simulink model "PEMFuelCellSystem_Cathode_cEGR_ExternalMembraneHumidifier_v01"  (R2025b)
settings: Solver=VariableStepAuto  StartTime=0.0  StopTime=100  MaxStep=0.1  RelTol=1e-3  AbsTol=1e-3
model workspace (MAT data in the model file):
  Gas_properties_block = 'PEMFuelCellSystem_Before_v01/Anode_Hydrogen_BOP/Gas Mixture
Properties'
  Gas_properties_candidates : object (value not decoded)
  T_TLU = [223.15 228.15 233.15 238.15 243.15 248.15 253.15 258.15 263.15 268.15 272.66 273.15 ... (115 elements, 1x115)]
  air_control_min_current_A = 3.8
  anode_separator_D = 0.02
  anode_separator_T0 = 20
  anode_separator_area = 0.000314159265359
  anode_separator_dp_nominal = 0.0005
  anode_separator_extra_length = 0.04
  anode_separator_laminar_fraction = 0.001
  anode_separator_length = 0.12
  anode_separator_mdot_nominal = 0.01
  anode_separator_p0 = 0.101325
  anode_separator_roughness = 1.5e-05
  anode_tube_D = 0.02
  cathode_channel_dp_nominal_MPa = 0.0368422
  cathode_channel_flow_area_m2 = 0.00403764556423
  cathode_channel_laminar_fraction = 0.5
  cathode_channel_mdot_nominal_kg_s = 0.27182
  cathode_outlet_chamber_V = 0.2
  cathode_separator_D = 0.05
  cathode_separator_T0 = 20
  cathode_separator_area = 0.00407150407905
  cathode_separator_dp_nominal = 0.002
  cathode_separator_extra_length = 0.05
  cathode_separator_laminar_fraction = 0.001
  cathode_separator_length = 0.15
  cathode_separator_mdot_nominal = 0.40798
  cathode_separator_p0 = 0.101325
  cathode_separator_roughness = 1.5e-05
  cathode_tube_D = 0.05
  cegr_comp_map_t_denom_epsilon = 1e-09
  cegr_cond_tau = 1
  cegr_inlet_mixer_p0 = 0.101325
  cegr_outlet_chamber_p0 = 0.101325
  cegr_pipe_D = 0.072
  cegr_pipe_area = 0.00407150407905
  cegr_pipe_extra_length = 0.1
  cegr_pipe_length = 0.5
  cegr_pipe_p0 = 0.101325
  cegr_pipe_roughness = 1.5e-05
  cegr_valve_max_area = 0.001
  cegr_valve_open_min_area = 1e-10
  comp_inlet_mixer_V = 0.1
  comp_mdot_corr_TLU = [0 0 0 0 0 0.28 0.26 0.24 0.22 0.2 0.56 0.52 ... (15 elements, 5x3)]
  comp_p_ratio_TLU = [1 1.5 2 2.5 3]
  comp_rpm_TLU = [0 50000 80000]
  coolant_num_layers = 20
  coolant_num_passes = 12
  coolant_tube_D = 0.05
  coolant_w_channels = 1
  drive_cycle_current = [0 0 100 100]
  drive_cycle_power = [0 0 40 40]
  drive_cycle_time = [0 0.5 60.5 600]
  drive_cycle_voltage = [427.6 427.6 410 410]
  env_RH = 0.5
  env_T = 20
  env_p = 0.101325
  env_pSat_H2O = 0.00233931818334
  env_yH20 = 0.0115436377169
  env_yO2 = 0.21
  exhaust_bp_valve_control_Ki_area_per_MPa_s = 0.002
  exhaust_bp_valve_max_area = 0.00134
  exhaust_bp_valve_open_min_area = 1e-10
  focused_anode_boundary_T_C = 20
  focused_anode_feed_p_MPa_abs = 0.3
  focused_anode_inlet_mdot_kg_s = 0.008
  focused_anode_inlet_p_MPa_abs = 0.161325
  focused_anode_outlet_p_MPa_abs = 0.101325
  focused_anode_pipe_area = 0.00246300864041
  focused_anode_pipe_extra_length = 0.1
  focused_anode_pipe_length = 1
  focused_anode_pipe_roughness = 1.5e-05
  focused_anode_yH2 = 0.9997
  focused_cathode_inlet_temperature_C = 58.9
  focused_stack_temperature_C = 80
  humidifier_bypass_mode : string (value not decoded)
  intercooler_Dh = 0.05
  intercooler_T0 = 20
  intercooler_area = 0.00785398163397
  intercooler_cond_tau = 1
  intercooler_dp_nominal = 0.005
  intercooler_extra_length = 0.05
  intercooler_laminar_fraction = 0.001
  intercooler_length = 0.25
  intercooler_mdot_nominal = 0.40798
  intercooler_p0 = 0.101325
  intercooler_roughness = 1.5e-05
  membrane_humidifier_dry_area_m2 = 0.01
  membrane_humidifier_dry_extra_length_m = 0.1
  membrane_humidifier_dry_hydraulic_diameter_m = 0.05
  membrane_humidifier_dry_length_m = 1
  membrane_humidifier_dry_roughness_m = 1.5e-05
  membrane_humidifier_heat_conductivity_W_per_m_K = 5
  membrane_humidifier_temperature_transfer_time_constant_s = 0.2
  membrane_humidifier_water_transfer_conductance_kg_s_Pa = 1e-08
  membrane_humidifier_water_transfer_time_constant_s = 0.5
  membrane_humidifier_wet_area_m2 = 0.01
  membrane_humidifier_wet_extra_length_m = 0.1
  membrane_humidifier_wet_hydraulic_diameter_m = 0.05
  membrane_humidifier_wet_length_m = 1
  membrane_humidifier_wet_roughness_m = 1.5e-05
  pSat_H2O_TLU = [0.0039376926592 0.00720321689378 0.0128411282011 0.0223441068076 0.0380050105363 0.0632733889962 0.103238678713 0.165273175188 0.259872929049 0.401739659013 0.586936061043 0.611151401419 ... (115 elements, 1x115)]
  pSat_TLU = [3379.45709837 5023.40410987 1277.63968517 0.0039376926592 3379.45809837 5023.40510987 1277.64068517 0.00720321689378 3379.45909837 5023.40610987 1277.64168517 0.0128411282011 ... (460 elements, 4x115)]
  radiator_H = 0.5
  radiator_L = 1
  radiator_N_fins = 12000
  radiator_N_tubes = 25
  radiator_W = 0.025
  radiator_air_area_fins = 11.5625
  radiator_air_area_primary = 1.223125
  radiator_cp = 910
  radiator_eta_fin = 0.7
  radiator_fin_spacing = 0.002
  radiator_gap_H = 0.0192708333333
  radiator_rho = 2700
  radiator_t_wall = 0.0001
  radiator_tube_H = 0.0015
  radiator_tube_Leq = 2.5
  routeA_air_control_mode_id = 2
  routeA_air_pid_Ki = 0.5
  routeA_air_pid_Kp = 5
  routeA_anode_inlet_pressure_MPa_abs = 0.161325
  routeA_anode_purge_enable = 1
  routeA_anode_purge_off_n2_mole_fraction = 0.1
  routeA_anode_purge_on_n2_mole_fraction = 0.5
  routeA_anode_recirculation_base_command = 0.2
  routeA_anode_recirculation_current_gain_A_inv = 0.00204081632653
  routeA_anode_rh_setpoint = 1
  routeA_backpressure_control_mode_id = 1
  routeA_cathode_humidifier_gain = 1
  routeA_cathode_rh_setpoint = 1
  routeA_cegr_enabled = 1
  routeA_cegr_valve_mode_id = 1
  routeA_command_profile = [0 0.5 60.5 600 0.101325 0.101325 0.101325 0.101325 20 20 20 20 ... (92 elements, 4x23)]
  routeA_command_profile_baseline = [0.101325 20 0.21 0.0115436377169 0.045 3 0.5 0.1613 1 1 0 70 ... (22 elements, 1x22)]
  routeA_command_profile_fields : string (value not decoded)
  routeA_command_profile_schema : string (value not decoded)
  routeA_current_default_ref_A = 28
  routeA_egr_control_Ki_area = 3.92699081699e-05
  routeA_egr_control_Kp_area = 0.000196349540849
  routeA_egr_control_mode_id = 1
  routeA_egr_target_input_mode_id = 1
  routeA_egr_valve_actuator_tau = 0.5
  routeA_egr_valve_area_direct = 3.92699081699e-06
  routeA_external_case_enabled = 0
  routeA_parameter_layer : string (value not decoded)
  routeA_stack_temperature_set_C = 80
  routeA_target_egr_ratio_comp_in = 0.02
  routeA_voltage_current_max_A = 392
  routeA_voltage_current_min_A = 0
  routeA_voltage_default_ref_V = 394.9
  routeA_voltage_pi_Ki = 0.05
  routeA_voltage_pi_Kp = 1
  separator_condensation_enabled = 1
  separator_l2_efficiency = 0.5
  separator_l2_source : string (value not decoded)
  stack_alpha = 1
  stack_area = 380
  stack_iL = 2.5
  stack_io = 2e-14
  stack_mea_cp = 870
  stack_mea_rho = 1800
  stack_num_cells = 606
  stack_num_channels = 8
  stack_t_gdl = 250
  stack_t_membrane = 125
  stack_w_channels = 1.16496474502
  tank_T = 20
  tank_V = 120
  tank_p = 70
  tank_yH2 = 0.9997
libraries: nesl_utility x57, FuelCell_lib x39, fl_lib x24, slpidlib x4
(part 4 of 6)

== system PEMFuelCellSystem_Cathode_cEGR_ExternalMembraneHumidifier_v01/Cathode_Air_Supply_and_cEGR/Cathode_Inlet_Instrumentation ==
  note: Function: in-line cathode inlet instrumentation.
      | Humidity Sensor W -> RH logging; Mass Flow Sensor M_i -> species mass-flow logging. No gas-state source is added here.
  Cathode_Inlet_EnergyFlow_Converter : nesl_utility/PS-Simulink Converter  Description=Convert cathode-inlet mixture energy flow [W] to the named inlet observability chain.  PhysicalDomain=network_engine_domain  SubClassName=ps_output  LeftPortType=input  RightPortType=output  PseudoPeriodic=off  Frequencies=[]  VectorFormat=inherit  Unit=W  AffineConversion=off
  Cathode_Inlet_Humidity_Sensor_FC : FuelCell_lib/sensors/Composition and Humidity Sensor (FC)
      settings: InternalSimscapePortConfiguration="{\"Bottom\":[],\"Left\":[{\"id\":\"A\",\"label\":\"A\",\"type\":\"FuelCell.FuelCell\"}],\"Right\":[{\"id\":\"x_i\",\"label\":\"x_i\",\"type\":\"output\"},{\"id\":\"y_i\",\"label\":\"y_i\",\"type\":\"output\"},{\"id\":\"W\",\"label\":\"W\",\"type\":\"output\"}],\"Top\":[]}"
  Cathode_Inlet_MassFraction_Converter : nesl_utility/PS-Simulink Converter  Description=Convert cathode-inlet sensor mass fractions to the named inlet observability chain.  PhysicalDomain=network_engine_domain  SubClassName=ps_output  LeftPortType=input  RightPortType=output  PseudoPeriodic=off  Frequencies=[]  VectorFormat=inherit  Unit=1  AffineConversion=off
  Cathode_Inlet_Mass_Flow_Sensor_FC : FuelCell_lib/sensors/Mass Flow Rate Sensor (FC)
      settings: InternalSimscapePortConfiguration="{\"Bottom\":[],\"Left\":[{\"id\":\"A\",\"label\":\"A\",\"type\":\"FuelCell.FuelCell\"}],\"Right\":[{\"id\":\"M\",\"label\":\"M\",\"type\":\"output\"},{\"id\":\"Phi_out\",\"label\":\"Phi\",\"type\":\"output\"},{\"id\":\"M_i\",\"label\":\"M_i\",\"type\":\"output\"},{\"id\":\"B\",\"label\":\"B\",\"type\":\"FuelCell.FuelCell\"}],\"Top\":[]}"
  Cathode_Inlet_Mdot_Converter : nesl_utility/PS-Simulink Converter  Description=Convert cathode-inlet total mass flow [kg/s] to the named inlet observability chain.  PhysicalDomain=network_engine_domain  SubClassName=ps_output  LeftPortType=input  RightPortType=output  PseudoPeriodic=off  Frequencies=[]  VectorFormat=inherit  Unit=kg/s  AffineConversion=off
  Cathode_Inlet_MoleFraction_Converter : nesl_utility/PS-Simulink Converter  Description=Convert cathode-inlet sensor mole fractions to the named inlet observability chain.  PhysicalDomain=network_engine_domain  SubClassName=ps_output  LeftPortType=input  RightPortType=output  PseudoPeriodic=off  Frequencies=[]  VectorFormat=inherit  Unit=1  AffineConversion=off
  Inlet_Result_Observability : Subsystem  Description=Records cathode-inlet relative humidity and species mass-flow vector for the V-SH result contract.
  cathode_air_from_bop : PMIOPort  Side=Left
  cathode_air_to_stack : PMIOPort  Port=2  Side=Right
  wires:
  Cathode_Inlet_MassFraction_Converter/1 -> Inlet_Result_Observability/1(inlet_mass_fraction)  "routeA_xi_ca_in_sensor"
  Cathode_Inlet_MoleFraction_Converter/1 -> Inlet_Result_Observability/2(inlet_mole_fraction)  "routeA_yi_ca_in_sensor"
  Cathode_Inlet_Mdot_Converter/1 -> Inlet_Result_Observability/3(inlet_mdot_kg_s)  "routeA_mdot_ca_in"
  Cathode_Inlet_EnergyFlow_Converter/1 -> Inlet_Result_Observability/4(inlet_energy_flow_W)  "routeA_energy_flow_ca_in_W"
  connections:
  Cathode_Inlet_Mass_Flow_Sensor_FC/RConn2 -- Cathode_Inlet_EnergyFlow_Converter/LConn1
  Cathode_Inlet_Humidity_Sensor_FC/RConn2 -- Cathode_Inlet_MoleFraction_Converter/LConn1
  Cathode_Inlet_Humidity_Sensor_FC/LConn1 -- Cathode_Inlet_Mass_Flow_Sensor_FC/LConn1 -- cathode_air_from_bop/RConn1
  Cathode_Inlet_Mass_Flow_Sensor_FC/RConn3 -- Inlet_Result_Observability/LConn2
  Cathode_Inlet_Mass_Flow_Sensor_FC/RConn1 -- Cathode_Inlet_Mdot_Converter/LConn1
  Cathode_Inlet_Humidity_Sensor_FC/RConn3 -- Inlet_Result_Observability/LConn1
  Cathode_Inlet_Humidity_Sensor_FC/RConn1 -- Cathode_Inlet_MassFraction_Converter/LConn1
  Cathode_Inlet_Mass_Flow_Sensor_FC/RConn4 -- cathode_air_to_stack/RConn1

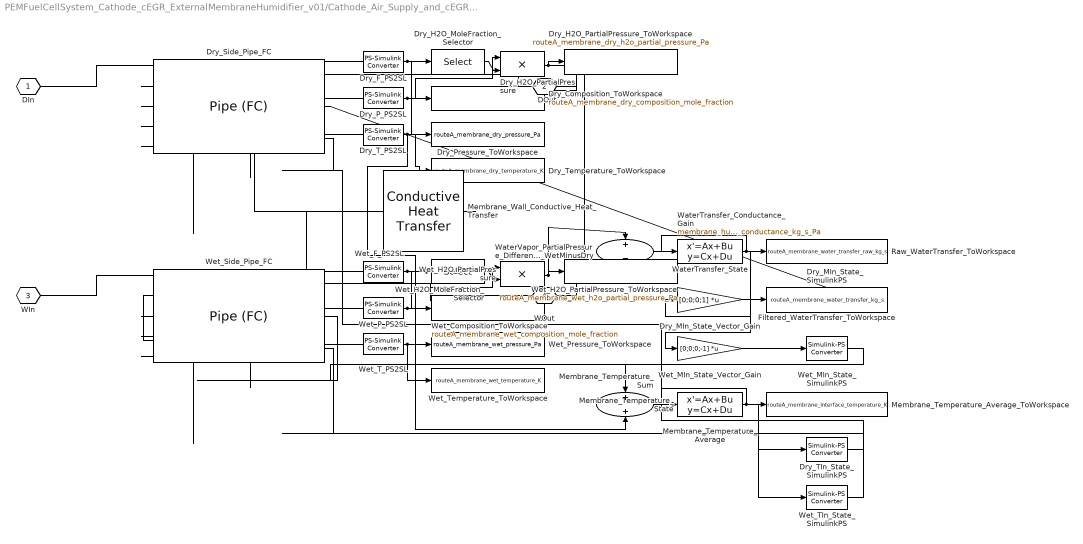
== system PEMFuelCellSystem_Cathode_cEGR_ExternalMembraneHumidifier_v01/Cathode_Air_Supply_and_cEGR/Cathode_Membrane_Humidifier ==
  Dry_Composition_ToWorkspace : ToWorkspace  VariableName=routeA_membrane_dry_composition_mole_fraction  SaveFormat=Structure With Time  SampleTime=-1
  Dry_F_PS2SL : nesl_utility/PS-Simulink Converter  PhysicalDomain=network_engine_domain  SubClassName=ps_output  LeftPortType=input  RightPortType=output  PseudoPeriodic=off  Frequencies=[]  VectorFormat=inherit  Unit=1  AffineConversion=off
  Dry_H2O_MoleFraction_Selector : Selector  InputPortWidth=4  IndexOptions=Index vector (dialog)  Indices=4  OutputSizes=1
  Dry_H2O_PartialPressure : Product  Inputs=**
  Dry_H2O_PartialPressure_ToWorkspace : ToWorkspace  VariableName=routeA_membrane_dry_h2o_partial_pressure_Pa  SaveFormat=Structure With Time  SampleTime=-1
  Dry_MIn_State_SimulinkPS : nesl_utility/Simulink-PS Converter  PhysicalDomain=network_engine_domain  SubClassName=ps_input  LeftPortType=input  RightPortType=output  PseudoPeriodic=off  Frequencies=[]  NoiseDistribution=none  NoiseParameters=[]  Unit=kg/s  AffineConversion=off  FilteringAndDerivatives=provide  SimscapeFilterOrder=1  InputFilterTimeConstant=0.001  UdotUserProvided=0
  Dry_MIn_State_Vector_Gain : Gain  Gain=[0;0;0;1]  Multiplication=Matrix(K*u)
  Dry_P_PS2SL : nesl_utility/PS-Simulink Converter  PhysicalDomain=network_engine_domain  SubClassName=ps_output  LeftPortType=input  RightPortType=output  PseudoPeriodic=off  Frequencies=[]  VectorFormat=inherit  Unit=Pa  AffineConversion=off
  Dry_Pressure_ToWorkspace : ToWorkspace  VariableName=routeA_membrane_dry_pressure_Pa  SaveFormat=Structure With Time  SampleTime=-1
  Dry_Side_Pipe_FC : FuelCell_lib/elements/Pipe (FC)  length=membrane_humidifier_dry_length_m m  area=membrane_humidifier_dry_area_m2 m^2  Dh=membrane_humidifier_dry_hydraulic_diameter_m m  extra_length=membrane_humidifier_dry_extra_length_m m  roughness=membrane_humidifier_dry_roughness_m m  Re_lam=2000  Re_tur=4000  shape_factor=64  Nu_lam=3.66  tau_c=cegr_cond_tau s  isCond=[0;0;0;0]  volMeas=true  compMeas=FuelCell.enum.Composition.Mole  p0=env_p MPa  T0=focused_cathode_inlet_temperature_C degC  comp=FuelCell.enum.Composition.Mole  y0=[1-env_yO2-env_yH20; env_yO2; 0; env_yH20]  x0=[1;0;0;0]
      settings: InternalSimscapePortConfiguration="{\"Bottom\":[{\"id\":\"MIn\",\"label\":\"M_in\",\"type\":\"input\"},{\"id\":\"TIn\",\"label\":\"T_in\",\"type\":\"input\"}],\"Left\":[{\"id\":\"A\",\"label\":\"A\",\"type\":\"FuelCell.FuelCell\"},{\"id\":\"H\",\"label\":\"H\",\"type\":\"foundation.thermal.thermal\"}],\"Right\":[{\"id\":\"B\",\"label\":\"B\",\"type\":\"FuelCell.FuelCell\"}],\"Top\":[{\"id\":\"F\",\"label\":\"F\",\"type\":\"output\"},{\"id\":\"p\",\"label\":\"p\",\"type\":\"output\"},{\"id\":\"T\",\"label\":\"T\",\"type\":\"output\"}]}"
  Dry_TIn_State_SimulinkPS : nesl_utility/Simulink-PS Converter  PhysicalDomain=network_engine_domain  SubClassName=ps_input  LeftPortType=input  RightPortType=output  PseudoPeriodic=off  Frequencies=[]  NoiseDistribution=none  NoiseParameters=[]  Unit=K  AffineConversion=off  FilteringAndDerivatives=provide  SimscapeFilterOrder=1  InputFilterTimeConstant=0.001  UdotUserProvided=0
  Dry_T_PS2SL : nesl_utility/PS-Simulink Converter  PhysicalDomain=network_engine_domain  SubClassName=ps_output  LeftPortType=input  RightPortType=output  PseudoPeriodic=off  Frequencies=[]  VectorFormat=inherit  Unit=K  AffineConversion=off
  Dry_Temperature_ToWorkspace : ToWorkspace  VariableName=routeA_membrane_dry_temperature_K  SaveFormat=Structure With Time  SampleTime=-1
  Filtered_WaterTransfer_ToWorkspace : ToWorkspace  VariableName=routeA_membrane_water_transfer_kg_s  SaveFormat=Structure With Time  SampleTime=-1
  Membrane_Temperature_Average : Gain  Gain=0.5
  Membrane_Temperature_Average_ToWorkspace : ToWorkspace  VariableName=routeA_membrane_interface_temperature_K  SaveFormat=Structure With Time  SampleTime=-1
  Membrane_Temperature_State : StateSpace  A=-1/membrane_humidifier_temperature_transfer_time_constant_s  B=1/membrane_humidifier_temperature_transfer_time_constant_s  D=0  InitialCondition=env_T+273.15
  Membrane_Temperature_Sum : Sum
  Membrane_Wall_Conductive_Heat_Transfer : fl_lib/Thermal/Thermal Elements/Conductive Heat Transfer  thermal_type=foundation.enum.ConstantVariableTabulated.Constant  wall_geometry=foundation.enum.ConductionWallGeometry.Planar  area=1 m^2  thickness=1 m  d_in=0.05 m  d_out=0.1 m  L=1 m  th_cond_min=10 W/(K*m)  th_cond=membrane_humidifier_heat_conductivity_W_per_m_K W/(K*m)  th_cond_TLU=[413, 401, 392, 383, 371, 357, 342] W/(K*m)  temp_TLU=[200, 273, 400, 600, 800, 1000, 1200] K  T_specify=off  T_priority=None  T=0 K  T_nominal_specify=off  T_nominal_value=1  T_nominal_unit=K  Q_specify=off  Q_priority=None  Q=0 W  Q_nominal_specify=off  Q_nominal_value=1  Q_nominal_unit=W
  Raw_WaterTransfer_ToWorkspace : ToWorkspace  VariableName=routeA_membrane_water_transfer_raw_kg_s  SaveFormat=Structure With Time  SampleTime=-1
  WaterTransfer_Conductance_Gain : Gain  Gain=membrane_humidifier_water_transfer_conductance_kg_s_Pa
  WaterTransfer_State : StateSpace  A=-1/membrane_humidifier_water_transfer_time_constant_s  B=1/membrane_humidifier_water_transfer_time_constant_s  D=0  InitialCondition=0
  WaterVapor_PartialPressure_Difference_WetMinusDry : Sum  Inputs=+-
  Wet_Composition_ToWorkspace : ToWorkspace  VariableName=routeA_membrane_wet_composition_mole_fraction  SaveFormat=Structure With Time  SampleTime=-1
  Wet_F_PS2SL : nesl_utility/PS-Simulink Converter  PhysicalDomain=network_engine_domain  SubClassName=ps_output  LeftPortType=input  RightPortType=output  PseudoPeriodic=off  Frequencies=[]  VectorFormat=inherit  Unit=1  AffineConversion=off
  Wet_H2O_MoleFraction_Selector : Selector  InputPortWidth=4  IndexOptions=Index vector (dialog)  Indices=4  OutputSizes=1
  Wet_H2O_PartialPressure : Product  Inputs=**
  Wet_H2O_PartialPressure_ToWorkspace : ToWorkspace  VariableName=routeA_membrane_wet_h2o_partial_pressure_Pa  SaveFormat=Structure With Time  SampleTime=-1
  Wet_MIn_State_SimulinkPS : nesl_utility/Simulink-PS Converter  PhysicalDomain=network_engine_domain  SubClassName=ps_input  LeftPortType=input  RightPortType=output  PseudoPeriodic=off  Frequencies=[]  NoiseDistribution=none  NoiseParameters=[]  Unit=kg/s  AffineConversion=off  FilteringAndDerivatives=provide  SimscapeFilterOrder=1  InputFilterTimeConstant=0.001  UdotUserProvided=0
  Wet_MIn_State_Vector_Gain : Gain  Gain=[0;0;0;-1]  Multiplication=Matrix(K*u)
  Wet_P_PS2SL : nesl_utility/PS-Simulink Converter  PhysicalDomain=network_engine_domain  SubClassName=ps_output  LeftPortType=input  RightPortType=output  PseudoPeriodic=off  Frequencies=[]  VectorFormat=inherit  Unit=Pa  AffineConversion=off
  Wet_Pressure_ToWorkspace : ToWorkspace  VariableName=routeA_membrane_wet_pressure_Pa  SaveFormat=Structure With Time  SampleTime=-1
  Wet_Side_Pipe_FC : FuelCell_lib/elements/Pipe (FC)  length=membrane_humidifier_wet_length_m m  area=membrane_humidifier_wet_area_m2 m^2  Dh=membrane_humidifier_wet_hydraulic_diameter_m m  extra_length=membrane_humidifier_wet_extra_length_m m  roughness=membrane_humidifier_wet_roughness_m m  Re_lam=2000  Re_tur=4000  shape_factor=64  Nu_lam=3.66  tau_c=cegr_cond_tau s  isCond=[0;0;0;0]  volMeas=true  compMeas=FuelCell.enum.Composition.Mole  p0=cegr_outlet_chamber_p0 MPa  T0=env_T degC  comp=FuelCell.enum.Composition.Mole  y0=[1-env_yO2-env_yH20; env_yO2; 0; env_yH20]  x0=[1-env_yO2-env_yH20; env_yO2; 0; env_yH20]
      settings: InternalSimscapePortConfiguration="{\"Bottom\":[{\"id\":\"MIn\",\"label\":\"M_in\",\"type\":\"input\"},{\"id\":\"TIn\",\"label\":\"T_in\",\"type\":\"input\"}],\"Left\":[{\"id\":\"A\",\"label\":\"A\",\"type\":\"FuelCell.FuelCell\"},{\"id\":\"H\",\"label\":\"H\",\"type\":\"foundation.thermal.thermal\"}],\"Right\":[{\"id\":\"B\",\"label\":\"B\",\"type\":\"FuelCell.FuelCell\"}],\"Top\":[{\"id\":\"F\",\"label\":\"F\",\"type\":\"output\"},{\"id\":\"p\",\"label\":\"p\",\"type\":\"output\"},{\"id\":\"T\",\"label\":\"T\",\"type\":\"output\"}]}"
  Wet_TIn_State_SimulinkPS : nesl_utility/Simulink-PS Converter  PhysicalDomain=network_engine_domain  SubClassName=ps_input  LeftPortType=input  RightPortType=output  PseudoPeriodic=off  Frequencies=[]  NoiseDistribution=none  NoiseParameters=[]  Unit=K  AffineConversion=off  FilteringAndDerivatives=provide  SimscapeFilterOrder=1  InputFilterTimeConstant=0.001  UdotUserProvided=0
  Wet_T_PS2SL : nesl_utility/PS-Simulink Converter  PhysicalDomain=network_engine_domain  SubClassName=ps_output  LeftPortType=input  RightPortType=output  PseudoPeriodic=off  Frequencies=[]  VectorFormat=inherit  Unit=K  AffineConversion=off
  Wet_Temperature_ToWorkspace : ToWorkspace  VariableName=routeA_membrane_wet_temperature_K  SaveFormat=Structure With Time  SampleTime=-1
  DIn : PMIOPort  Side=Left
  DOut : PMIOPort  Port=2  Side=Right
  WIn : PMIOPort  Port=3  Side=Left
  WOut : PMIOPort  Port=4  Side=Right
  wires:
  Dry_F_PS2SL/1 -> Dry_H2O_MoleFraction_Selector/1, Dry_Composition_ToWorkspace/1
  Dry_P_PS2SL/1 -> Dry_H2O_PartialPressure/1, Dry_Pressure_ToWorkspace/1
  Dry_T_PS2SL/1 -> Dry_Temperature_ToWorkspace/1, Membrane_Temperature_Sum/1
  Dry_H2O_MoleFraction_Selector/1 -> Dry_H2O_PartialPressure/2
  Dry_H2O_PartialPressure/1 -> Dry_H2O_PartialPressure_ToWorkspace/1, WaterVapor_PartialPressure_Difference_WetMinusDry/2
  Wet_F_PS2SL/1 -> Wet_H2O_MoleFraction_Selector/1, Wet_Composition_ToWorkspace/1
  Wet_P_PS2SL/1 -> Wet_Pressure_ToWorkspace/1, Wet_H2O_PartialPressure/1
  Wet_T_PS2SL/1 -> Wet_Temperature_ToWorkspace/1, Membrane_Temperature_Sum/2
  Wet_H2O_MoleFraction_Selector/1 -> Wet_H2O_PartialPressure/2
  Wet_H2O_PartialPressure/1 -> Wet_H2O_PartialPressure_ToWorkspace/1, WaterVapor_PartialPressure_Difference_WetMinusDry/1
  WaterVapor_PartialPressure_Difference_WetMinusDry/1 -> WaterTransfer_Conductance_Gain/1
  Membrane_Temperature_Sum/1 -> Membrane_Temperature_Average/1
  Dry_MIn_State_Vector_Gain/1 -> Dry_MIn_State_SimulinkPS/1
  Wet_MIn_State_Vector_Gain/1 -> Wet_MIn_State_SimulinkPS/1
  WaterTransfer_State/1 -> Filtered_WaterTransfer_ToWorkspace/1, Dry_MIn_State_Vector_Gain/1, Wet_MIn_State_Vector_Gain/1
  Membrane_Temperature_State/1 -> Dry_TIn_State_SimulinkPS/1, Wet_TIn_State_SimulinkPS/1
  WaterTransfer_Conductance_Gain/1 -> WaterTransfer_State/1, Raw_WaterTransfer_ToWorkspace/1
  Membrane_Temperature_Average/1 -> Membrane_Temperature_State/1, Membrane_Temperature_Average_ToWorkspace/1
  connections:
  DIn/RConn1 -- Dry_Side_Pipe_FC/LConn1
  Dry_Side_Pipe_FC/RConn1 -- DOut/RConn1
  WIn/RConn1 -- Wet_Side_Pipe_FC/LConn1
  Wet_Side_Pipe_FC/RConn1 -- WOut/RConn1
  Membrane_Wall_Conductive_Heat_Transfer/RConn1 -- Wet_Side_Pipe_FC/LConn2
  Dry_Side_Pipe_FC/LConn3 -- Dry_F_PS2SL/LConn1
  Dry_Side_Pipe_FC/LConn4 -- Dry_P_PS2SL/LConn1
  Dry_Side_Pipe_FC/LConn5 -- Dry_T_PS2SL/LConn1
  Wet_Side_Pipe_FC/LConn3 -- Wet_F_PS2SL/LConn1
  Wet_Side_Pipe_FC/LConn4 -- Wet_P_PS2SL/LConn1
  Wet_Side_Pipe_FC/LConn5 -- Wet_T_PS2SL/LConn1
  Dry_Side_Pipe_FC/LConn2 -- Membrane_Wall_Conductive_Heat_Transfer/LConn1
  Wet_TIn_State_SimulinkPS/RConn1 -- Wet_Side_Pipe_FC/RConn3
  Wet_MIn_State_SimulinkPS/RConn1 -- Wet_Side_Pipe_FC/RConn2
  Dry_TIn_State_SimulinkPS/RConn1 -- Dry_Side_Pipe_FC/RConn3
  Dry_MIn_State_SimulinkPS/RConn1 -- Dry_Side_Pipe_FC/RConn2

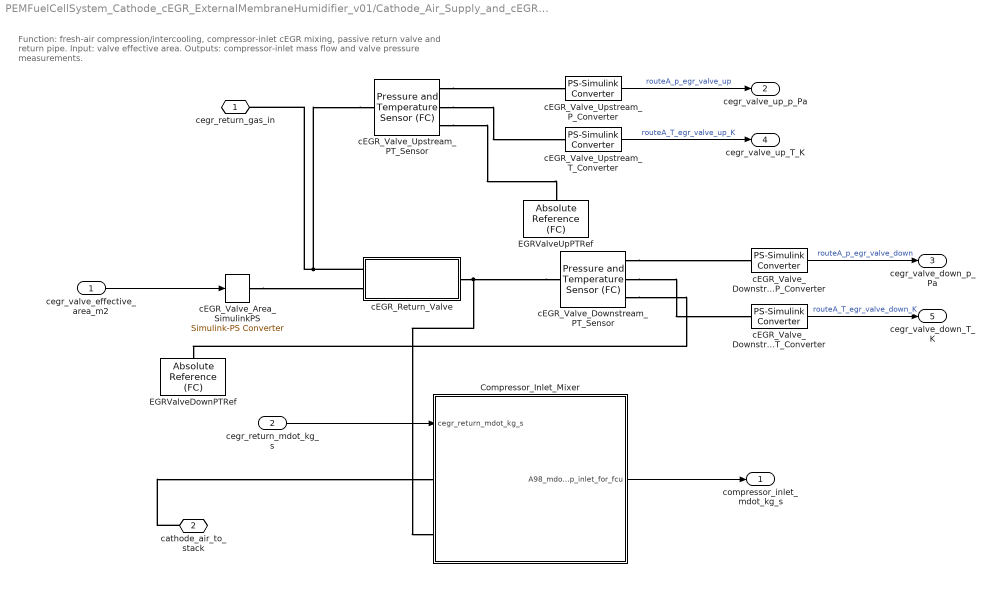
== system PEMFuelCellSystem_Cathode_cEGR_ExternalMembraneHumidifier_v01/Cathode_Air_Supply_and_cEGR/Fresh_Air_Compression_and_cEGR ==
  note: Function: fresh-air compression/intercooling, compressor-inlet cEGR mixing, passive return valve and return pipe.
      | Input: valve effective area. Outputs: compressor-inlet mass flow and valve pressure measurements.
  cegr_valve_effective_area_m2 : Inport
  cegr_return_mdot_kg_s : Inport  Port=2
  Compressor_Inlet_Mixer : Subsystem  Tag=PublishSubsystem  Description=Fresh-air boundary, compressor and intercooler path with compressor-inlet cEGR mixing. External humidifier injection is disabled for V-SH.
      mask Display:
      | plot(0, 0)
      | plot(100, 100)
      | 
      | n = 80;
      | r1 = 15;
      | r2 = 30;
      | 
      | plot(cos(linspace(0, 2*pi, n))*r1 + 65, sin(linspace(0, 2*pi, n))*r1 + 50)
      | plot(cos(linspace(0, 2*pi, n))*r2 + 65, sin(linspace(0, 2*pi, n))*r2 + 50)
      | 
      | plot([65 30 30 42], [80 80 70 70])
  EGRValveDownPTRef : FuelCell_lib/elements/Absolute Reference (FC)
      settings: InternalSimscapePortConfiguration="{\"Bottom\":[],\"Left\":[{\"id\":\"A\",\"label\":\"\",\"type\":\"FuelCell.FuelCell\"}],\"Right\":[],\"Top\":[]}"
  EGRValveUpPTRef : FuelCell_lib/elements/Absolute Reference (FC)
      settings: InternalSimscapePortConfiguration="{\"Bottom\":[],\"Left\":[{\"id\":\"A\",\"label\":\"\",\"type\":\"FuelCell.FuelCell\"}],\"Right\":[],\"Top\":[]}"
  cEGR_Return_Valve : Subsystem  Variant=on
  cEGR_Valve_Area_SimulinkPS : nesl_utility/Simulink-PS Converter  PhysicalDomain=network_engine_domain  SubClassName=ps_input  LeftPortType=input  RightPortType=output  PseudoPeriodic=off  Frequencies=[]  NoiseDistribution=none  NoiseParameters=[]  Unit=m^2  AffineConversion=off  FilteringAndDerivatives=provide  SimscapeFilterOrder=1  InputFilterTimeConstant=0.001  UdotUserProvided=0
  cEGR_Valve_Downstream_PT_Sensor : FuelCell_lib/sensors/Pressure and Temperature Sensor (FC)
      settings: InternalSimscapePortConfiguration="{\"Bottom\":[],\"Left\":[{\"id\":\"A\",\"label\":\"A\",\"type\":\"FuelCell.FuelCell\"}],\"Right\":[{\"id\":\"P\",\"label\":\"P\",\"type\":\"output\"},{\"id\":\"T\",\"label\":\"T\",\"type\":\"output\"},{\"id\":\"B\",\"label\":\"B\",\"type\":\"FuelCell.FuelCell\"}],\"Top\":[]}"
  cEGR_Valve_Downstream_P_Converter : nesl_utility/PS-Simulink Converter  PhysicalDomain=network_engine_domain  SubClassName=ps_output  LeftPortType=input  RightPortType=output  PseudoPeriodic=off  Frequencies=[]  VectorFormat=inherit  Unit=inherit  AffineConversion=off
  cEGR_Valve_Downstream_T_Converter : nesl_utility/PS-Simulink Converter  Description=Convert measured valve-downstream gas temperature from the FC physical-signal domain to a named Simulink diagnostic.  PhysicalDomain=network_engine_domain  SubClassName=ps_output  LeftPortType=input  RightPortType=output  PseudoPeriodic=off  Frequencies=[]  VectorFormat=inherit  Unit=K  AffineConversion=off
  cEGR_Valve_Upstream_PT_Sensor : FuelCell_lib/sensors/Pressure and Temperature Sensor (FC)
      settings: InternalSimscapePortConfiguration="{\"Bottom\":[],\"Left\":[{\"id\":\"A\",\"label\":\"A\",\"type\":\"FuelCell.FuelCell\"}],\"Right\":[{\"id\":\"P\",\"label\":\"P\",\"type\":\"output\"},{\"id\":\"T\",\"label\":\"T\",\"type\":\"output\"},{\"id\":\"B\",\"label\":\"B\",\"type\":\"FuelCell.FuelCell\"}],\"Top\":[]}"
  cEGR_Valve_Upstream_P_Converter : nesl_utility/PS-Simulink Converter  PhysicalDomain=network_engine_domain  SubClassName=ps_output  LeftPortType=input  RightPortType=output  PseudoPeriodic=off  Frequencies=[]  VectorFormat=inherit  Unit=inherit  AffineConversion=off
  cEGR_Valve_Upstream_T_Converter : nesl_utility/PS-Simulink Converter  Description=Convert measured valve-upstream gas temperature from the FC physical-signal domain to a named Simulink diagnostic.  PhysicalDomain=network_engine_domain  SubClassName=ps_output  LeftPortType=input  RightPortType=output  PseudoPeriodic=off  Frequencies=[]  VectorFormat=inherit  Unit=K  AffineConversion=off
  cegr_return_gas_in : PMIOPort  Side=Left
  cathode_air_to_stack : PMIOPort  Port=2  Side=Right
  compressor_inlet_mdot_kg_s : Outport
  cegr_valve_up_p_Pa : Outport  Port=2
  cegr_valve_down_p_Pa : Outport  Port=3
  cegr_valve_up_T_K : Outport  Description=Valve-upstream gas temperature [K], measured against the FC absolute reference.  Port=4
  cegr_valve_down_T_K : Outport  Description=Valve-downstream gas temperature [K], measured against the FC absolute reference.  Port=5
  wires:
  cegr_valve_effective_area_m2/1 -> cEGR_Valve_Area_SimulinkPS/1
  cEGR_Valve_Downstream_P_Converter/1 -> cegr_valve_down_p_Pa/1  "routeA_p_egr_valve_down"
  Compressor_Inlet_Mixer/1(A98_mdot_comp_inlet_for_fcu) -> compressor_inlet_mdot_kg_s/1
  cegr_return_mdot_kg_s/1 -> Compressor_Inlet_Mixer/1(cegr_return_mdot_kg_s)
  cEGR_Valve_Downstream_T_Converter/1 -> cegr_valve_down_T_K/1  "routeA_T_egr_valve_down_K"
  cEGR_Valve_Upstream_P_Converter/1 -> cegr_valve_up_p_Pa/1  "routeA_p_egr_valve_up"
  cEGR_Valve_Upstream_T_Converter/1 -> cegr_valve_up_T_K/1  "routeA_T_egr_valve_up_K"
  connections:
  cEGR_Valve_Area_SimulinkPS/RConn1 -- cEGR_Return_Valve/LConn2
  cEGR_Valve_Upstream_PT_Sensor/RConn3 -- EGRValveUpPTRef/LConn1
  cEGR_Valve_Upstream_PT_Sensor/RConn2 -- cEGR_Valve_Upstream_T_Converter/LConn1
  cEGR_Valve_Upstream_PT_Sensor/RConn1 -- cEGR_Valve_Upstream_P_Converter/LConn1
  cEGR_Valve_Downstream_PT_Sensor/LConn1 -- cEGR_Return_Valve/RConn1 -- Compressor_Inlet_Mixer/LConn2
  cathode_air_to_stack/RConn1 -- Compressor_Inlet_Mixer/LConn1
  cEGR_Valve_Downstream_PT_Sensor/RConn1 -- cEGR_Valve_Downstream_P_Converter/LConn1
  cEGR_Valve_Downstream_PT_Sensor/RConn2 -- cEGR_Valve_Downstream_T_Converter/LConn1
  cEGR_Valve_Upstream_PT_Sensor/LConn1 -- cEGR_Return_Valve/LConn1 -- cegr_return_gas_in/RConn1
  cEGR_Valve_Downstream_PT_Sensor/RConn3 -- EGRValveDownPTRef/LConn1

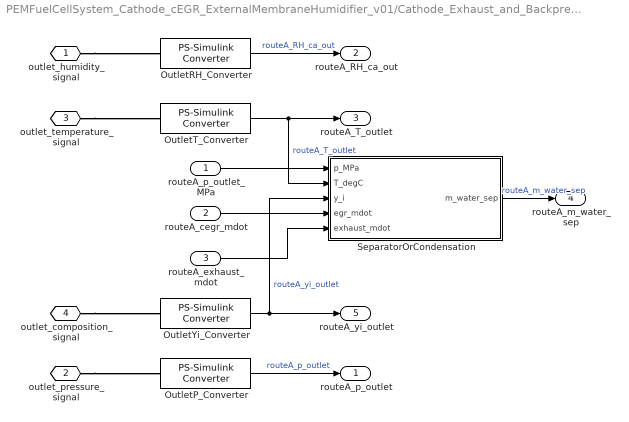
== system PEMFuelCellSystem_Cathode_cEGR_ExternalMembraneHumidifier_v01/Cathode_Exhaust_and_Backpressure/CathodeOutlet_Observability ==
  routeA_p_outlet_MPa : Inport
  routeA_cegr_mdot : Inport  Port=2
  routeA_exhaust_mdot : Inport  Port=3
  OutletP_Converter : nesl_utility/PS-Simulink Converter  Description=Convert cathode outlet pressure physical signal to Simulink output.  PhysicalDomain=network_engine_domain  SubClassName=ps_output  LeftPortType=input  RightPortType=output  PseudoPeriodic=off  Frequencies=[]  VectorFormat=inherit  Unit=inherit  AffineConversion=off
  OutletRH_Converter : nesl_utility/PS-Simulink Converter  Description=Convert cathode outlet relative-humidity physical signal to Simulink output.  PhysicalDomain=network_engine_domain  SubClassName=ps_output  LeftPortType=input  RightPortType=output  PseudoPeriodic=off  Frequencies=[]  VectorFormat=inherit  Unit=inherit  AffineConversion=off
  OutletT_Converter : nesl_utility/PS-Simulink Converter  Description=Convert cathode outlet temperature physical signal to Simulink output.  PhysicalDomain=network_engine_domain  SubClassName=ps_output  LeftPortType=input  RightPortType=output  PseudoPeriodic=off  Frequencies=[]  VectorFormat=inherit  Unit=inherit  AffineConversion=off
  OutletYi_Converter : nesl_utility/PS-Simulink Converter  Description=Convert cathode outlet composition physical signal to Simulink output.  PhysicalDomain=network_engine_domain  SubClassName=ps_output  LeftPortType=input  RightPortType=output  PseudoPeriodic=off  Frequencies=[]  VectorFormat=inherit  Unit=inherit  AffineConversion=off
  SeparatorOrCondensation : MATLAB Function  Description=L2 gas-phase water-separation audit observer; does not alter gas composition.  TreatAsAtomicUnit=on
  outlet_humidity_signal : PMIOPort  Side=Left
  outlet_pressure_signal : PMIOPort  Port=2  Side=Left
  outlet_temperature_signal : PMIOPort  Port=3  Side=Left
  outlet_composition_signal : PMIOPort  Port=4  Side=Left
  routeA_p_outlet : Outport
  routeA_RH_ca_out : Outport  Port=2
  routeA_T_outlet : Outport  Port=3
  routeA_m_water_sep : Outport  Port=4
  routeA_yi_outlet : Outport  Port=5
  wires:
  routeA_cegr_mdot/1 -> SeparatorOrCondensation/4(egr_mdot)
  routeA_p_outlet_MPa/1 -> SeparatorOrCondensation/1(p_MPa)
  routeA_exhaust_mdot/1 -> SeparatorOrCondensation/5(exhaust_mdot)
  OutletT_Converter/1 -> SeparatorOrCondensation/2(T_degC), routeA_T_outlet/1  "routeA_T_outlet"
  OutletRH_Converter/1 -> routeA_RH_ca_out/1  "routeA_RH_ca_out"
  OutletYi_Converter/1 -> SeparatorOrCondensation/3(y_i), routeA_yi_outlet/1  "routeA_yi_outlet"
  OutletP_Converter/1 -> routeA_p_outlet/1  "routeA_p_outlet"
  SeparatorOrCondensation/1(m_water_sep) -> routeA_m_water_sep/1  "routeA_m_water_sep"
  connections:
  outlet_pressure_signal/RConn1 -- OutletP_Converter/LConn1
  outlet_composition_signal/RConn1 -- OutletYi_Converter/LConn1
  outlet_temperature_signal/RConn1 -- OutletT_Converter/LConn1
  outlet_humidity_signal/RConn1 -- OutletRH_Converter/LConn1

== system PEMFuelCellSystem_Cathode_cEGR_ExternalMembraneHumidifier_v01/Cathode_Exhaust_and_Backpressure/Exhaust_Environment_Boundary ==
  Environment : FuelCell_lib/elements/Reservoir (FC)  constCond=true  p0=env_p MPa  T0=env_T degC  comp=FuelCell.enum.Composition.Mole  y0=[1-env_yO2-env_yH20; env_yO2; 0; env_yH20]  x0=[1; 0; 0; 0]  area=pi*cathode_tube_D^2/4 m^2
      settings: InternalSimscapePortConfiguration="{\"Bottom\":[],\"Left\":[],\"Right\":[],\"Top\":[{\"id\":\"A\",\"label\":\"A\",\"type\":\"FuelCell.FuelCell\"}]}"
  C : PMIOPort  Side=Left
  connections:
  C/RConn1 -- Environment/LConn1

== system PEMFuelCellSystem_Cathode_cEGR_ExternalMembraneHumidifier_v01/Cathode_Exhaust_and_Backpressure/Exhaust_Flow_and_Composition_Diagnostics ==
  ca_out_mass_fraction : Inport
  ca_out_mole_fraction : Inport  Port=2
  cegr_energy_flow_W : Inport  Port=3
  cegr_species_mdot_kg_s : Inport  Port=4
  exhaust_energy_flow_W : Inport  Port=5
  exhaust_species_mdot_kg_s : Inport  Port=6
  Cathode_Outlet_MassFraction_ToWorkspace : ToWorkspace  VariableName=routeA_xi_ca_out_sensor_ts  SaveFormat=Structure With Time
      settings: Description=Cathode-outlet sensor mass-fraction vector [N2/O2/H2/H2O].
  Cathode_Outlet_MoleFraction_ToWorkspace : ToWorkspace  VariableName=routeA_yi_ca_out_sensor_ts  SaveFormat=Structure With Time
      settings: Description=Cathode-outlet sensor mole-fraction vector [N2/O2/H2/H2O].
  Exhaust_EnergyFlow_ToWorkspace : ToWorkspace  VariableName=routeA_exhaust_energy_flow_W_ts  SaveFormat=Structure With Time
      settings: Description=Exhaust mixture energy flow [W], positive from sensor A to B.
  Exhaust_SpeciesMdot_ToWorkspace : ToWorkspace  VariableName=routeA_exhaust_species_mdot_kg_s_ts  SaveFormat=Structure With Time
      settings: Description=Exhaust species mass-flow vector [kg/s], positive from sensor A to B.
  cEGR_EnergyFlow_ToWorkspace : ToWorkspace  VariableName=routeA_cegr_energy_flow_W_ts  SaveFormat=Structure With Time
      settings: Description=cEGR return mixture energy flow [W], positive from sensor A to B.
  cEGR_SpeciesMdot_ToWorkspace : ToWorkspace  VariableName=routeA_cegr_species_mdot_kg_s_ts  SaveFormat=Structure With Time
      settings: Description=cEGR return species mass-flow vector [kg/s], positive from sensor A to B.
  wires:
  ca_out_mole_fraction/1 -> Cathode_Outlet_MoleFraction_ToWorkspace/1  "routeA_yi_ca_out_sensor"
  exhaust_species_mdot_kg_s/1 -> Exhaust_SpeciesMdot_ToWorkspace/1  "routeA_exhaust_species_mdot_kg_s"
  exhaust_energy_flow_W/1 -> Exhaust_EnergyFlow_ToWorkspace/1  "routeA_exhaust_energy_flow_W"
  ca_out_mass_fraction/1 -> Cathode_Outlet_MassFraction_ToWorkspace/1  "routeA_xi_ca_out_sensor"
  cegr_species_mdot_kg_s/1 -> cEGR_SpeciesMdot_ToWorkspace/1  "routeA_cegr_species_mdot_kg_s"
  cegr_energy_flow_W/1 -> cEGR_EnergyFlow_ToWorkspace/1  "routeA_cegr_energy_flow_W"

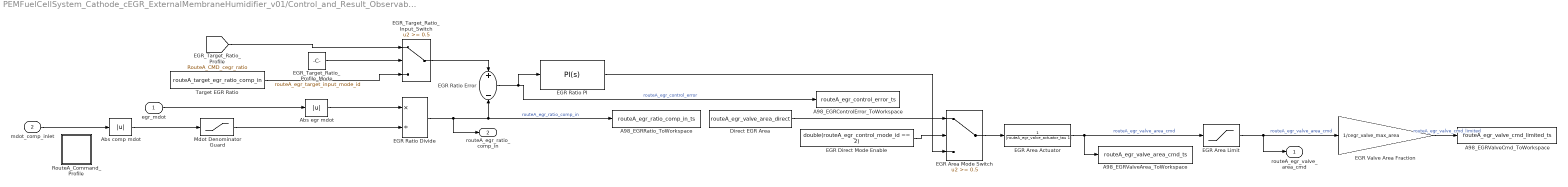
== system PEMFuelCellSystem_Cathode_cEGR_ExternalMembraneHumidifier_v01/Control_and_Result_Observability/Cathode_cEGR_Control ==
  egr_mdot : Inport
  mdot_comp_inlet : Inport  Port=2
  A98_EGRControlError_ToWorkspace : ToWorkspace  VariableName=routeA_egr_control_error_ts  SaveFormat=Structure With Time  SampleTime=-1
  A98_EGRRatio_ToWorkspace : ToWorkspace  VariableName=routeA_egr_ratio_comp_in_ts  SaveFormat=Structure With Time  SampleTime=-1
  A98_EGRValveArea_ToWorkspace : ToWorkspace  VariableName=routeA_egr_valve_area_cmd_ts  SaveFormat=Structure With Time  SampleTime=-1
  A98_EGRValveCmd_ToWorkspace : ToWorkspace  VariableName=routeA_egr_valve_cmd_limited_ts  SaveFormat=Structure With Time  SampleTime=-1
  Abs comp mdot : Abs  ZeroCross=off  SaturateOnIntegerOverflow=off
  Abs egr mdot : Abs  ZeroCross=off  SaturateOnIntegerOverflow=off
  Direct EGR Area : Constant  Value=routeA_egr_valve_area_direct
  EGR Area Actuator : TransferFcn  Denominator=[routeA_egr_valve_actuator_tau 1]
  EGR Area Limit : Saturate  UpperLimit=cegr_valve_max_area  LowerLimit=cegr_valve_open_min_area
  EGR Area Mode Switch : Switch  Threshold=0.5  SaturateOnIntegerOverflow=off  InputSameDT=off
  EGR Direct Mode Enable : Constant  Value=double(routeA_egr_control_mode_id == 2)
  EGR Ratio Divide : Product  Inputs=*/
  EGR Ratio Error : Sum  Inputs=+-
  EGR Ratio PI : slpidlib/PID Controller  Controller=PI  Form=Parallel  TimeDomain=Continuous-time  UseExternalTs=off  SampleTime=-1  IntegratorMethod=Forward Euler  FilterMethod=Forward Euler  ControllerParametersSource=internal  P=routeA_egr_control_Kp_area  I=routeA_egr_control_Ki_area  UseKiTs=off  D=0  UseExternalDerivativeSource=off  N=100  UseFilter=on  TunerSelectOption=Transfer Function Based (PID Tuner App)  ZeroCross=off  InitialConditionSource=internal  InitialConditionForIntegrator=cegr_valve_open_min_area  InitialConditionForFilter=0  DifferentiatorICPrevScaledInput=0  ExternalReset=none  TrackingMode=off  Kt=1  LimitOutput=on  SatLimitsSource=internal  UpperSaturationLimit=cegr_valve_max_area  LowerSaturationLimit=cegr_valve_open_min_area  LinearizeAsGain=on  AntiWindupMode=none  Kb=1  LimitIntegrator=off  UpperIntegratorSaturationLimit=inf  LowerIntegratorSaturationLimit=-inf  POutMin=[]  POutMax=[]  IOutMin=[]  IOutMax=[]  DOutMin=[]  DOutMax=[]  NOutMin=[]  NOutMax=[]  SumOutMin=[]  SumOutMax=[]  SaturationOutMin=[]  SaturationOutMax=[]  PParamMin=[]  PParamMax=[]  IParamMin=[]  IParamMax=[]  DParamMin=[]  DParamMax=[]  NParamMin=[]  NParamMax=[]  KbParamMin=[]  KbParamMax=[]  KtParamMin=[]  KtParamMax=[]  KbOutMin=[]  KbOutMax=[]  KtOutMin=[]  KtOutMax=[]  IntegratorOutMin=[]  IntegratorOutMax=[]  FilterOutMin=[]  FilterOutMax=[]  SumI1OutMin=[]  SumI1OutMax=[]  SumI2OutMin=[]  SumI2OutMax=[]  SumI3OutMin=[]  SumI3OutMax=[]  SumI4OutMin=[]  SumI4OutMax=[]  SumDOutMin=[]  SumDOutMax=[]  DifferentiatorOutMin=[]  DifferentiatorOutMax=[]  FilterDiffOutCoefMin=[]  FilterDiffOutCoefMax=[]  ReciprocalOutMin=[]  ReciprocalOutMax=[]  SumDenOutMin=[]  SumDenOutMax=[]  SumNumOutMin=[]  SumNumOutMax=[]  DivideOutMin=[]  DivideOutMax=[]  UdiffTsProdOutMin=[]  UdiffTsProdOutMax=[]  NTsProdOutMin=[]  NTsProdOutMax=[]  UintegralTsProdOutMin=[]  UintegralTsProdOutMax=[]  UngainTsProdOutMin=[]  UngainTsProdOutMax=[]  ClampingZeroOutDataTypeStr=Inherit: Inherit via back propagation  ClampingZeroOutMin=[]  ClampingZeroOutMax=[]  FilterDenConstantOutDataTypeStr=Inherit: Inherit via back propagation  FilterDenConstantOutMin=[]  FilterDenConstantOutMax=[]  PCopyOutDataTypeStr=Inherit: Inherit via back propagation  PCopyOutMin=[]  PCopyOutMax=[]  NCopyOutDataTypeStr=Inherit: Inherit via back propagation  NCopyOutMin=[]  NCopyOutMax=[]  IntegratorContinuousStateAttributes=''  IntegratorStateMustResolveToSignalObject=off  IntegratorRTWStateStorageClass=Auto  FilterContinuousStateAttributes=''  FilterStateMustResolveToSignalObject=off  FilterRTWStateStorageClass=Auto  ParallelPVariant=InternalParameters  IdealPVariant=Disabled  IVariant=InternalParameters  DVariant=Disabled  IntegratorVariant=Continuous  SatVariant=Enabled  AWVariant=Passthrough  PCopyVariant=Disabled  TRVariant=Disabled  FdbkBlocksVariant=Forward  IdealPFdbkVariant=Disabled  SatFdbkVariant=Disabled  DerivativeFilterVariant=Disabled  NVariant=Disabled  NCopyVariant=Disabled_SignalSpec  FilterICVariant=Disabled  IntegratorICVariant=InternalICs  ExternalResetVariant=Disabled  TRSumVariant=Passthrough  SumFdbkVariant=Disabled  SumVariant=Sum_PI  TsampFilterVariant=InternalTs  TsampNgainVariant=Passthrough  TsampIntegralVariant=Disabled_SignalSpec  ExternalSaturationOutDataTypeStr=Inherit: Same as second input  DerivativeSourceVariant=Disabled  PreIntVariant=InternalPreInt
  EGR Valve Area Fraction : Gain  Gain=1/cegr_valve_max_area
  EGR_Target_Ratio_Input_Switch : Switch  Threshold=0.5
  EGR_Target_Ratio_Profile_Mode : Constant  Value=routeA_egr_target_input_mode_id
  Mdot Denominator Guard : Saturate  UpperLimit=inf  LowerLimit=1e-6  ZeroCross=off
  RouteA_Command_Profile : Subsystem
  Target EGR Ratio : Constant  Value=routeA_target_egr_ratio_comp_in
  routeA_egr_valve_area_cmd : Outport
  routeA_egr_ratio_comp_in : Outport  Port=2
  wires:
  mdot_comp_inlet/1 -> Abs comp mdot/1
  EGR Valve Area Fraction/1 -> A98_EGRValveCmd_ToWorkspace/1  "routeA_egr_valve_cmd_limited"
  Abs comp mdot/1 -> Mdot Denominator Guard/1
  egr_mdot/1 -> Abs egr mdot/1
  Target EGR Ratio/1 -> EGR_Target_Ratio_Input_Switch/3
  Abs egr mdot/1 -> EGR Ratio Divide/1
  Mdot Denominator Guard/1 -> EGR Ratio Divide/2
  EGR Ratio Error/1 -> A98_EGRControlError_ToWorkspace/1, EGR Ratio PI/1  "routeA_egr_control_error"
  EGR Ratio Divide/1 -> A98_EGRRatio_ToWorkspace/1, EGR Ratio Error/2, routeA_egr_ratio_comp_in/1  "routeA_egr_ratio_comp_in"
  Direct EGR Area/1 -> EGR Area Mode Switch/1
  EGR Direct Mode Enable/1 -> EGR Area Mode Switch/2
  EGR Ratio PI/1 -> EGR Area Mode Switch/3
  EGR Area Mode Switch/1 -> EGR Area Actuator/1
  EGR Area Actuator/1 -> A98_EGRValveArea_ToWorkspace/1, EGR Area Limit/1  "routeA_egr_valve_area_cmd"
  EGR Area Limit/1 -> routeA_egr_valve_area_cmd/1, EGR Valve Area Fraction/1  "routeA_egr_valve_area_cmd"
  EGR_Target_Ratio_Profile_Mode/1 -> EGR_Target_Ratio_Input_Switch/2
  EGR_Target_Ratio_Input_Switch/1 -> EGR Ratio Error/1
  [RouteA_CMD_cegr_ratio] -> EGR_Target_Ratio_Input_Switch/1

== system PEMFuelCellSystem_Cathode_cEGR_ExternalMembraneHumidifier_v01/Control_and_Result_Observability/Electrical_Load_Boundary ==
  Controlled Current Source : fl_lib/Electrical/Electrical Sources/Controlled Current Source
  Electrical Reference : fl_lib/Electrical/Electrical Elements/Electrical Reference
  Inputs : Subsystem  Variant=on  VariantControlMode=label  LabelModeActiveChoice=Voltage
      settings: PortSchema="{\"entries\":[{\"content\":{\"sides\":[{\"content\":{\"connectorIds\":[\"LConn1\"]},\"type\":\"ConnectorPlacement.EquallySpacedRectSide\",\"uuid\":\"316ab41f-9548-4c29-941b-82cd3006a9cc\"},{\"content\":{\"connectorIds\":[],\"side\":\"RIGHT\"},\"type\":\"ConnectorPlacement.EquallySpacedRectSide\",\"uuid\":\"21ddf6a1-5f8a-47a4-ab15-3c27c3a556ce\"},{\"content\":{\"connectorIds\":[\"LConn2\"],\"side\":\"TOP\"},\"type\":\"ConnectorPlacement.EquallySpacedRectSide\",\"uuid\":\"59191a52-f145-4ac2-9cf2-0e0b54b3d2a8\"}]},\"type\":\"ConnectorPlacement.EquallySpacedConnector\",\"uuid\":\"e8f988fd-b412-4b1a-aaea-374cf82170cc\"}],\"packageUris\":[\"http://schema.mathworks.com/mf0/Connector/R2020b\"],\"version\":\"1.0\"}"
      mask Display:
      | blk = get_param(gcb, 'CompiledActiveChoiceBlock');
      | eval(get_param(blk, 'MaskDisplay'))
  Voltage Sensor : fl_lib/Electrical/Electrical Sensors/Voltage Sensor
  - : PMIOPort  Side=Right
  + : PMIOPort  Port=2  Side=Right
  connections:
  Electrical Reference/LConn1 -- Controlled Current Source/LConn1 -- -/RConn1 -- Voltage Sensor/RConn2
  +/RConn1 -- Voltage Sensor/LConn1 -- Controlled Current Source/RConn2
  Voltage Sensor/RConn1 -- Inputs/LConn2
  Inputs/LConn1 -- Controlled Current Source/RConn1

== system PEMFuelCellSystem_Cathode_cEGR_ExternalMembraneHumidifier_v01/Control_and_Result_Observability/Stack_Performance_Measurements ==
  Focused_Zero_HeatFlow : Constant  Value=0
  stack_power_kW_gain : Gain  Gain=1e-3
  stack_power_mux : Mux  Inputs=2
  stack_power_product : Product
  stack_current_A : Outport
  stack_voltage_V : Outport  Port=2
  stack_power_kW : Outport  Port=3
  stack_temperature_C : Outport  Port=4
  wires:
  [i_stack] -> stack_current_A/1, stack_power_product/1
  Focused_Zero_HeatFlow/1 -> [Q_stack]
  stack_power_mux/1 -> stack_power_kW/1
  [Q_stack] -> stack_power_mux/2
  stack_power_kW_gain/1 -> stack_power_mux/1
  stack_power_product/1 -> stack_power_kW_gain/1
  [v_stack] -> stack_voltage_V/1, stack_power_product/2
  [T_stack] -> stack_temperature_C/1

== system PEMFuelCellSystem_Cathode_cEGR_ExternalMembraneHumidifier_v01/PEMFC_Stack_Core/Anode_Gas_Channels ==
  Anode : FuelCell_lib/elements/Constant Volume Chamber (FC)  V0=stack_w_channels^2 * stack_num_channels * stack_num_cells * sqrt(stack_area) cm^3  num_ports=foundation.enum.num_ports.three  area_A=stack_w_channels^2 * stack_num_channels * stack_num_cells cm^2  area_B=stack_w_channels^2 * stack_num_channels * stack_num_cells cm^2  area_C=stack_w_channels^2 * stack_num_channels * stack_num_cells cm^2  area_D=0.01 m^2  cond_spec=FuelCell.enum.ChamberCondSpec.Enabled  tau_c=1e-3 s  is_cond=[0; 0; 0; 0]  out_comp=FuelCell.enum.Composition.Mass  p0=env_p MPa  T0=env_T degC  comp=FuelCell.enum.Composition.Mole  y0=[0; 0; 1; 0]  x0=[1; 0; 0; 0]
      settings: InternalSimscapePortConfiguration="{\"Bottom\":[{\"id\":\"H\",\"label\":\"H\",\"type\":\"foundation.thermal.thermal\"}],\"Left\":[{\"id\":\"MIn\",\"label\":\"MIn\",\"type\":\"input\"},{\"id\":\"TIn\",\"label\":\"TIn\",\"type\":\"input\"}],\"Right\":[{\"id\":\"pC\",\"label\":\"p\",\"type\":\"output\"},{\"id\":\"TC\",\"label\":\"T\",\"type\":\"output\"},{\"id\":\"xC_i\",\"label\":\"x_i\",\"type\":\"output\"}],\"Top\":[{\"id\":\"A\",\"label\":\"A\",\"type\":\"FuelCell.FuelCell\"},{\"id\":\"B\",\"label\":\"B\",\"type\":\"FuelCell.FuelCell\"},{\"id\":\"C\",\"label\":\"C\",\"type\":\"FuelCell.FuelCell\"}]}"
  A : PMIOPort  Side=Right
  Min : PMIOPort  Port=2  Side=Right
  Tin : PMIOPort  Port=3  Side=Right
  H : PMIOPort  Port=4  Side=Right
  B : PMIOPort  Port=5  Side=Left
  C : PMIOPort  Port=6  Side=Left
  xi : PMIOPort  Port=7  Side=Left
  connections:
  B/RConn1 -- Anode/LConn4
  Min/RConn1 -- Anode/LConn1
  Tin/RConn1 -- Anode/LConn2
  xi/RConn1 -- Anode/RConn3
  Anode/LConn5 -- C/RConn1
  A/RConn1 -- Anode/LConn3
  H/RConn1 -- Anode/RConn4

== system PEMFuelCellSystem_Cathode_cEGR_ExternalMembraneHumidifier_v01/PEMFC_Stack_Core/Cathode_Gas_Channels ==
  Cathode : FuelCell_lib/elements/Constant Volume Chamber (FC)  V0=stack_w_channels^2 * stack_num_channels * stack_num_cells * sqrt(stack_area) cm^3  num_ports=foundation.enum.num_ports.three  area_A=stack_w_channels^2 * stack_num_channels * stack_num_cells cm^2  area_B=stack_w_channels^2 * stack_num_channels * stack_num_cells cm^2  area_C=stack_w_channels^2 * stack_num_channels * stack_num_cells cm^2  area_D=0.01 m^2  cond_spec=FuelCell.enum.ChamberCondSpec.Enabled  tau_c=1e-3 s  is_cond=[0; 0; 0; 0]  out_comp=FuelCell.enum.Composition.Mass  p0=env_p MPa  T0=env_T degC  comp=FuelCell.enum.Composition.Mole  y0=[1-env_yO2-env_yH20; env_yO2; 0; env_yH20]  x0=[1; 0; 0; 0]
      settings: InternalSimscapePortConfiguration="{\"Bottom\":[{\"id\":\"H\",\"label\":\"H\",\"type\":\"foundation.thermal.thermal\"}],\"Left\":[{\"id\":\"MIn\",\"label\":\"MIn\",\"type\":\"input\"},{\"id\":\"TIn\",\"label\":\"TIn\",\"type\":\"input\"}],\"Right\":[{\"id\":\"pC\",\"label\":\"p\",\"type\":\"output\"},{\"id\":\"TC\",\"label\":\"T\",\"type\":\"output\"},{\"id\":\"xC_i\",\"label\":\"x_i\",\"type\":\"output\"}],\"Top\":[{\"id\":\"A\",\"label\":\"A\",\"type\":\"FuelCell.FuelCell\"},{\"id\":\"B\",\"label\":\"B\",\"type\":\"FuelCell.FuelCell\"},{\"id\":\"C\",\"label\":\"C\",\"type\":\"FuelCell.FuelCell\"}]}"
  A : PMIOPort  Side=Right
  Min : PMIOPort  Port=2  Side=Right
  Tin : PMIOPort  Port=3  Side=Right
  H : PMIOPort  Port=4  Side=Right
  B : PMIOPort  Port=5  Side=Left
  C : PMIOPort  Port=6  Side=Left
  xi : PMIOPort  Port=7  Side=Left
  connections:
  B/RConn1 -- Cathode/LConn4
  Min/RConn1 -- Cathode/LConn1
  Tin/RConn1 -- Cathode/LConn2
  xi/RConn1 -- Cathode/RConn3
  H/RConn1 -- Cathode/RConn4
  Cathode/LConn5 -- C/RConn1
  A/RConn1 -- Cathode/LConn3
